simulink model "GradualClampTestslx"  (R2021b)
settings: Solver=FixedStepAuto  StartTime=0.0  StopTime=inf  RelTol=1e-3  EnableMultiTasking=on
libraries: vexarmcortexlib x23, simulink x8, vexcommonlib x2
settings Model: SimulationMode=external  NumberOfSteps=6  Creator=arago  LastModifiedBy=arago
settings DataIOCC: LimitDataPoints=on  SignalLoggingSaveFormat=ModelDataLogs  ReturnWorkspaceOutputs=off
settings OptimizationCC: ExpressionDepthLimit=2147483647  LifeSpan=Inf  MaxStackSize=64  EfficientTunableParamExpr=on
settings DebuggingCC: UnderspecifiedInitializationDetection=Classic  MergeDetectMultiDrivingBlocksExec=none  InheritedTsInSrcMsg=none  FcnCallInpInsideContextMsg=warning  UnconnectedInputMsg=none  UnconnectedOutputMsg=none  StateNameClashWarn=warning  SFUnexpectedBacktrackingDiag=warning  SFNoUnconditionalDefaultTransitionDiag=warning  SFExecutionAtInitializationDiag=none  SFMachineParentedDataDiag=warning  ArithmeticOperatorsInVariantConditions=warning
settings HardwareCC: ProdBitPerPointer=32  ProdBitPerSizeT=32  ProdBitPerPtrDiffT=32  ProdLargestAtomicInteger=Long  ProdLargestAtomicFloat=Double  ProdIntDivRoundTo=Undefined  ProdWordSize=32  ProdHWDeviceType=ARM Compatible->ARM Cortex
settings ModelReferenceCC: PropagateSignalLabelsOutOfModel=off
settings SFSimCC: MATLABDynamicMemAlloc=off  CustomCodeUndefinedFunction=UseInterfaceOnly
settings RTWCC: Description=Embedded Coder  SystemTargetFile=ert.tlc  HardwareBoard=ARM Cortex-based VEX Microcontroller  TemplateMakefile=ert_default_tmf  Toolchain=GNU Tools for VEX ARM Cortex
settings CodeAppCC: IgnoreCustomStorageClasses=off  CustomSymbolStrType=$N$R$M  StateflowObjectComments=on  InternalIdentifier=Classic
settings ERTTargetCC: CodeReplacementLibrary=GCC ARM Cortex-M3  MultiwordLength=2048  ConvertIfToSwitch=off  SuppressUnreachableDefaultCases=off

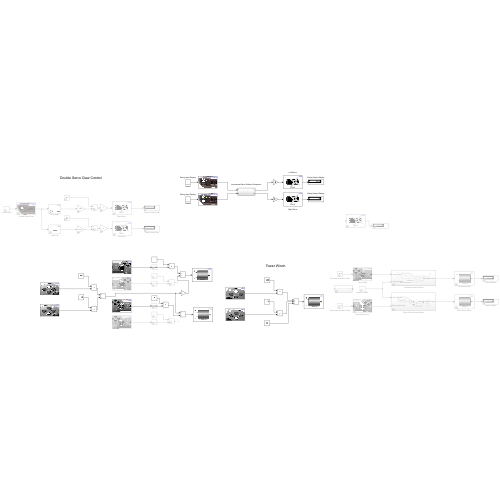
[thumbnail: Simulink's stored preview of the top-level diagram]
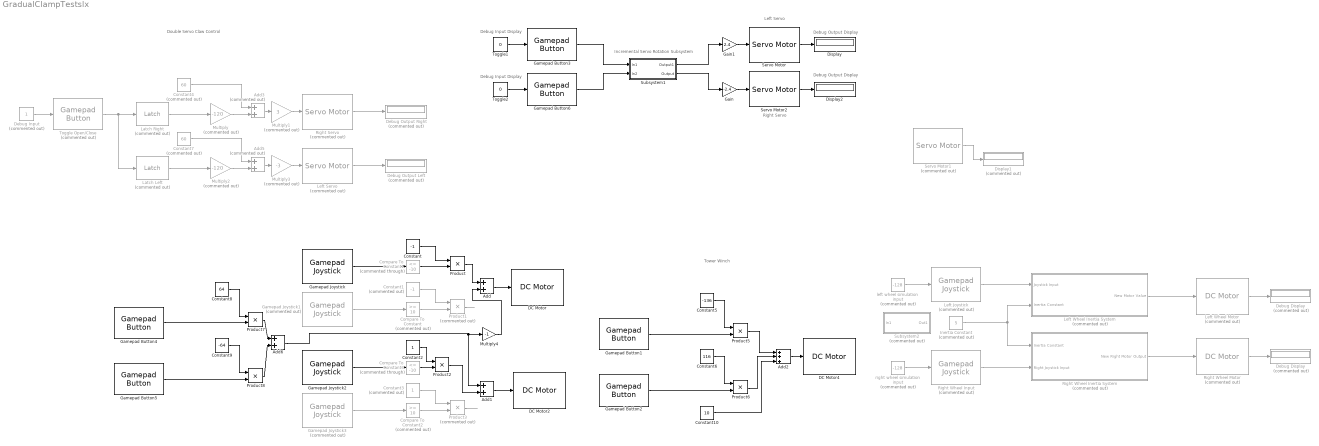
== system GradualClampTestslx ==
  note: Incremental Servo Rotation Subsystem
  note: Left Servo
  note: Double Servo Claw Control
  note: Tower Winch
  note: Right Servo
  note: Debug Output Display
  note: Debug Output Display
  note: Debug Input Display
  note: Debug Input Display
  " Debug Display" : Display  Commented=on
  Add : Sum
  Add1 : Sum
  Add2 : Sum  Inputs=+++
  Add3 : Sum  Commented=on
  Add5 : Sum  Commented=on
  Add6 : Sum
  Compare To Constant : simulink/Logic and Bit Operations/Compare To Constant  Commented=on  relop=>=  const=10  OutDataTypeStr=uint8
  Compare To Constant1 : simulink/Logic and Bit Operations/Compare To Constant  Commented=through  relop=<=  const=-10  OutDataTypeStr=uint8
  Compare To Constant2 : simulink/Logic and Bit Operations/Compare To Constant  Commented=on  relop=>=  const=10  OutDataTypeStr=uint8
  Compare To Constant3 : simulink/Logic and Bit Operations/Compare To Constant  Commented=through  relop=<=  const=-10  OutDataTypeStr=uint8
  Constant : Constant  Value=-1
  Constant1 : Constant  Commented=on  Value=-1
  Constant10 : Constant  Value=10
  Constant2 : Constant
  Constant3 : Constant  Commented=on
  Constant4 : Constant  Commented=on  Value=60
  Constant5 : Constant  Value=-136
  Constant6 : Constant  Value=116
  Constant7 : Constant  Commented=on  Value=60
  Constant8 : Constant  Value=64
  Constant9 : Constant  Value=-64
  DC Motor : vexarmcortexlib/Actuators/DC Motor  motor=2  scaleFactor=1/13.5  SimulationOut=off
      settings: SourceProductBaseCode=EC_VEX_MICRO
  DC Motor2 : vexarmcortexlib/Actuators/DC Motor  motor=3  scaleFactor=1/13.5  SimulationOut=off
      settings: SourceProductBaseCode=EC_VEX_MICRO
  DC Motor4 : vexarmcortexlib/Actuators/DC Motor  motor=6  scaleFactor=1/13.5  SimulationOut=off
      settings: SourceProductBaseCode=EC_VEX_MICRO
  Debug Display : Display  Commented=on
  Debug Input : Constant  Commented=on
      settings: OpenFcn=|
      | if strcmp('0',get_param(gcb, 'Value'))                        set_param(gcb, 'Value', '1');
      | else
      |             set_param(gcb, 'Value', '0');
      | end
  Debug Output Left : Display  Commented=on
  Debug Output Right : Display  Commented=on
  Display : Display
  Display1 : Display  Commented=on
  Display2 : Display
  Gain : Gain  Gain=-2.4
  Gain1 : Gain  Gain=2.4
  Gamepad Button1 : vexarmcortexlib/Gamepad/Gamepad Button  joystick=1  chan=8  button56=Up  button78=Up  SimulationIn=off  SampleTime=0.02
      settings: SourceProductBaseCode=EC_VEX_MICRO
  Gamepad Button2 : vexarmcortexlib/Gamepad/Gamepad Button  joystick=1  chan=8  button56=Up  button78=Down  SimulationIn=off  SampleTime=0.02
      settings: SourceProductBaseCode=EC_VEX_MICRO
  Gamepad Button3 : vexarmcortexlib/Gamepad/Gamepad Button  joystick=1  chan=6  button56=Up  button78=Down  SimulationIn=on  SampleTime=0.02
      settings: SourceProductBaseCode=EC_VEX_MICRO
  Gamepad Button4 : vexarmcortexlib/Gamepad/Gamepad Button  joystick=1  chan=7  button56=Up  button78=Up  SimulationIn=off  SampleTime=0.02
      settings: SourceProductBaseCode=EC_VEX_MICRO
  Gamepad Button5 : vexarmcortexlib/Gamepad/Gamepad Button  joystick=1  chan=7  button56=Up  button78=Down  SimulationIn=off  SampleTime=0.02
      settings: SourceProductBaseCode=EC_VEX_MICRO
  Gamepad Button6 : vexarmcortexlib/Gamepad/Gamepad Button  joystick=1  chan=6  button56=Down  button78=Down  SimulationIn=on  SampleTime=0.02
      settings: SourceProductBaseCode=EC_VEX_MICRO
  Gamepad Joystick : vexarmcortexlib/Gamepad/Gamepad Joystick  joystick=1  chan=2  SimulationIn=off  SampleTime=0.02
      settings: SourceProductBaseCode=EC_VEX_MICRO
  Gamepad Joystick1 : vexarmcortexlib/Gamepad/Gamepad Joystick  Commented=on  joystick=1  chan=2  SimulationIn=off  SampleTime=0.02
      settings: SourceProductBaseCode=EC_VEX_MICRO
  Gamepad Joystick2 : vexarmcortexlib/Gamepad/Gamepad Joystick  joystick=1  chan=3  SimulationIn=off  SampleTime=0.02
      settings: SourceProductBaseCode=EC_VEX_MICRO
  Gamepad Joystick3 : vexarmcortexlib/Gamepad/Gamepad Joystick  Commented=on  joystick=1  chan=3  SimulationIn=off  SampleTime=0.02
      settings: SourceProductBaseCode=EC_VEX_MICRO
  Inertia Constant : Constant  Commented=on  Value=5
  Latch Left : vexcommonlib/Latch  Commented=on  output0=off  BlockPlatform=vexarmcortex
      settings: SourceProductBaseCode=EC_VEX_MICRO,VEXV5
  Latch Right : vexcommonlib/Latch  Commented=on  output0=off  BlockPlatform=vexarmcortex
      settings: SourceProductBaseCode=EC_VEX_MICRO,VEXV5
  Left Joystick : vexarmcortexlib/Gamepad/Gamepad Joystick  Commented=on  joystick=1  chan=3  SimulationIn=on  SampleTime=0.02
      settings: SourceProductBaseCode=EC_VEX_MICRO
  Left Servo : vexarmcortexlib/Actuators/Servo Motor  Commented=on  motor=4  scaleFactor=60/127  SimulationOut=on
      settings: SourceProductBaseCode=EC_VEX_MICRO
  Left Wheel Inertia System : Subsystem  Commented=on
  Left Wheel Motor : vexarmcortexlib/Actuators/DC Motor  Commented=on  motor=2  scaleFactor=1/13.5  SimulationOut=on
      settings: SourceProductBaseCode=EC_VEX_MICRO
  Multiply : Gain  Commented=on  Gain=-120
  Multiply1 : Gain  Commented=on  Gain=3
  Multiply2 : Gain  Commented=on  Gain=-120
  Multiply3 : Gain  Commented=on  Gain=-3
  Multiply4 : Gain  Gain=-1
  Product{,2,5..8} (6 alike) : Product
  Product1 : Product  Commented=on
  Product3 : Product  Commented=on
  Right Servo : vexarmcortexlib/Actuators/Servo Motor  Commented=on  motor=5  scaleFactor=60/127  SimulationOut=on
      settings: SourceProductBaseCode=EC_VEX_MICRO
  Right Wheel Inertia System : Subsystem  Commented=on
  Right Wheel Input : vexarmcortexlib/Gamepad/Gamepad Joystick  Commented=on  joystick=1  chan=2  SimulationIn=on  SampleTime=0.02
      settings: SourceProductBaseCode=EC_VEX_MICRO
  Right Wheel Motor : vexarmcortexlib/Actuators/DC Motor  Commented=on  motor=3  scaleFactor=1/13.5  SimulationOut=on
      settings: SourceProductBaseCode=EC_VEX_MICRO
  Servo Motor : vexarmcortexlib/Actuators/Servo Motor  motor=5  scaleFactor=60/127  SimulationOut=on
      settings: SourceProductBaseCode=EC_VEX_MICRO
  Servo Motor1 : vexarmcortexlib/Actuators/Servo Motor  Commented=on  motor=5  scaleFactor=60/127  SimulationOut=on
      settings: SourceProductBaseCode=EC_VEX_MICRO
  Servo Motor2 : vexarmcortexlib/Actuators/Servo Motor  motor=4  scaleFactor=60/127  SimulationOut=on
      settings: SourceProductBaseCode=EC_VEX_MICRO
  Subsystem1 : Subsystem
  Subsystem2 : Subsystem  Commented=on
  Toggle Open/Close : vexarmcortexlib/Gamepad/Gamepad Button  Commented=on  joystick=1  chan=6  button56=Up  button78=Down  SimulationIn=on  SampleTime=0.02
      settings: SourceProductBaseCode=EC_VEX_MICRO
  Toggle1 : Constant  Value=0
      settings: OpenFcn=|
      | if strcmp('0',get_param(gcb, 'Value'))                        set_param(gcb, 'Value', '1');
      | else
      |             set_param(gcb, 'Value', '0');
      | end
  Toggle2 : Constant  Value=0
      settings: OpenFcn=|
      | if strcmp('0',get_param(gcb, 'Value'))                        set_param(gcb, 'Value', '1');
      | else
      |             set_param(gcb, 'Value', '0');
      | end
  left wheel simulation input : Constant  Commented=on  Value=-128  SampleTime=0.02
  right wheel simulation input : Constant  Commented=on  Value=-128  SampleTime=0.02
  wires:
  Gamepad Joystick1/1 -> Compare To Constant/1
  Gamepad Joystick/1 -> Compare To Constant1/1
  Compare To Constant/1 -> Product1/2
  Compare To Constant1/1 -> Product/2
  Constant/1 -> Product/1
  Constant1/1 -> Product1/1
  Constant2/1 -> Product2/1
  Constant3/1 -> Product3/1
  Gamepad Joystick2/1 -> Compare To Constant3/1
  Compare To Constant3/1 -> Product2/2
  Product3/1 -> ?
  Product2/1 -> Add1/2
  Compare To Constant2/1 -> Product3/2
  Gamepad Joystick3/1 -> Compare To Constant2/1
  Toggle Open/Close/1 -> Latch Left/1, Latch Right/1
  Latch Right/1 -> Multiply/1
  Constant4/1 -> Add3/1
  Gamepad Button1/1 -> Product5/2
  Constant5/1 -> Product5/1
  Product5/1 -> Add2/1
  Product6/1 -> Add2/2
  Constant6/1 -> Product6/1
  Gamepad Button2/1 -> Product6/2
  Add/1 -> DC Motor/1
  Product/1 -> Add/1
  Product1/1 -> ?
  Add1/1 -> DC Motor2/1
  Add2/1 -> DC Motor4/1
  Debug Input/1 -> Toggle Open/Close/1
  Servo Motor/1 -> Display/1
  Multiply/1 -> Add3/2
  Add3/1 -> Multiply1/1
  Toggle1/1 -> Gamepad Button3/1
  Gamepad Button3/1 -> Subsystem1/1(In1)
  Servo Motor1/1 -> Display1/1
  Constant7/1 -> Add5/1
  Multiply2/1 -> Add5/2
  Latch Left/1 -> Multiply2/1
  Servo Motor2/1 -> Display2/1
  Add5/1 -> Multiply3/1
  Add6/1 -> Multiply4/1, Add1/1
  Gamepad Button5/1 -> Product8/2
  Product7/1 -> Add6/1
  Product8/1 -> Add6/2
  Gamepad Button4/1 -> Product7/2
  Constant9/1 -> Product8/1
  Constant8/1 -> Product7/1
  Multiply4/1 -> Add/2
  Subsystem1/1(Output1) -> Gain1/1
  Subsystem1/2(Output) -> Gain/1
  Toggle2/1 -> Gamepad Button6/1
  Gamepad Button6/1 -> Subsystem1/2(In2)
  Left Wheel Motor/1 -> " Debug Display"/1
  right wheel simulation input/1 -> Right Wheel Input/1
  Right Wheel Inertia System/1(New Right Motor Output) -> Right Wheel Motor/1
  left wheel simulation input/1 -> Left Joystick/1
  Right Wheel Motor/1 -> Debug Display/1
  Left Wheel Inertia System/1(New Motor Value) -> Left Wheel Motor/1
  Right Wheel Input/1 -> Right Wheel Inertia System/2(Right Joystick Input)
  Inertia Constant/1 -> Right Wheel Inertia System/1(Inertia Constant), Left Wheel Inertia System/2(Inertia Constant)
  Left Joystick/1 -> Left Wheel Inertia System/1(Joystick Input)
  Gain/1 -> Servo Motor2/1
  Gain1/1 -> Servo Motor/1
  Right Servo/1 -> Debug Output Right/1
  Left Servo/1 -> Debug Output Left/1
  Multiply1/1 -> Right Servo/1
  Multiply3/1 -> Left Servo/1
  Constant10/1 -> Add2/3

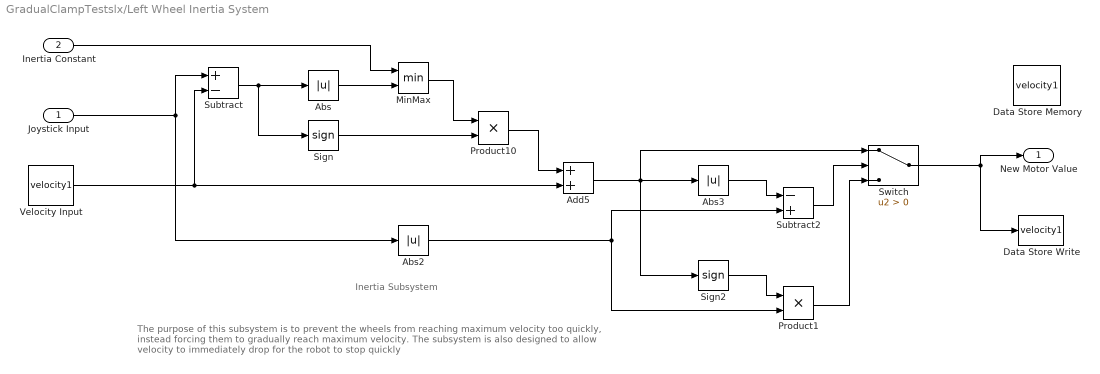
== system GradualClampTestslx/Left Wheel Inertia System ==
  note: The purpose of this subsystem is to prevent the wheels from reaching maximum velocity too quickly, instead forcing them to gradually reach maximum velocity. The subsystem is also designed to allow velocity to immediately drop for the robot to stop quickly
  note: Inertia Subsystem
  Joystick Input : Inport
  Inertia Constant : Inport  Port=2
  Abs : Abs
  Abs2 : Abs
  Abs3 : Abs
  Add5 : Sum
  Data Store Memory : DataStoreMemory  DataStoreName=velocity1  ReadBeforeWriteMsg=warning  WriteAfterWriteMsg=warning  WriteAfterReadMsg=warning  ShowAdditionalParam=off
  Data Store Write : DataStoreWrite  DataStoreName=velocity1  SampleTime=0.02  IndexOptions=Index vector (dialog)  Indices=1  OutputSizes=1
  MinMax : MinMax  Inputs=2
  Product1 : Product  RndMeth=Zero
  Product10 : Product  RndMeth=Zero
  Sign : Signum
  Sign2 : Signum
  Subtract : Sum  Inputs=+-
  Subtract2 : Sum  Inputs=-+
  Switch : Switch  Criteria=u2 > Threshold
  Velocity Input : DataStoreRead  DataStoreName=velocity1  SampleTime=0.02  IndexOptions=Index vector (dialog)  Indices=1  OutputSizes=1
  New Motor Value : Outport
  wires:
  Joystick Input/1 -> Subtract/1, Abs2/1
  Subtract/1 -> Sign/1, Abs/1
  Add5/1 -> Sign2/1, Switch/1, Abs3/1
  Abs/1 -> MinMax/2
  Sign/1 -> Product10/2
  Velocity Input/1 -> Subtract/2, Add5/2
  Abs2/1 -> Subtract2/2, Product1/2
  Product10/1 -> Add5/1
  Sign2/1 -> Product1/1
  MinMax/1 -> Product10/1
  Inertia Constant/1 -> MinMax/1
  Switch/1 -> New Motor Value/1, Data Store Write/1
  Subtract2/1 -> Switch/2
  Abs3/1 -> Subtract2/1
  Product1/1 -> Switch/3

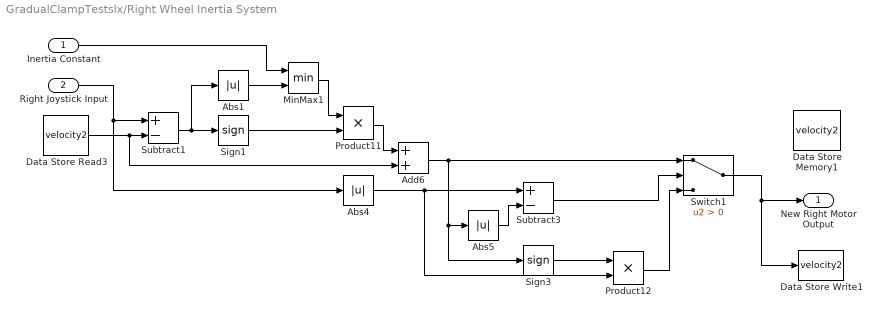
== system GradualClampTestslx/Right Wheel Inertia System ==
  Inertia Constant : Inport
  Right Joystick Input : Inport  Port=2
  Abs1 : Abs
  Abs4 : Abs
  Abs5 : Abs
  Add6 : Sum
  Data Store Memory1 : DataStoreMemory  DataStoreName=velocity2  ReadBeforeWriteMsg=warning  WriteAfterWriteMsg=warning  WriteAfterReadMsg=warning  ShowAdditionalParam=off
  Data Store Read3 : DataStoreRead  DataStoreName=velocity2  SampleTime=0.02  IndexOptions=Index vector (dialog)  Indices=1  OutputSizes=1
  Data Store Write1 : DataStoreWrite  DataStoreName=velocity2  SampleTime=0.02  IndexOptions=Index vector (dialog)  Indices=1  OutputSizes=1
  MinMax1 : MinMax  Inputs=2
  Product11 : Product  RndMeth=Zero
  Product12 : Product  RndMeth=Zero
  Sign1 : Signum
  Sign3 : Signum
  Subtract1 : Sum  Inputs=+-
  Subtract3 : Sum  Inputs=+-
  Switch1 : Switch  Criteria=u2 > Threshold
  New Right Motor Output : Outport
  wires:
  MinMax1/1 -> Product11/1
  Abs5/1 -> Subtract3/2
  Product11/1 -> Add6/1
  Abs4/1 -> Product12/2, Subtract3/1
  Abs1/1 -> MinMax1/2
  Subtract3/1 -> Switch1/2
  Subtract1/1 -> Abs1/1, Sign1/1
  Sign1/1 -> Product11/2
  Sign3/1 -> Product12/1
  Data Store Read3/1 -> Subtract1/2, Add6/2
  Add6/1 -> Abs5/1, Sign3/1, Switch1/1
  Right Joystick Input/1 -> Abs4/1, Subtract1/1
  Inertia Constant/1 -> MinMax1/1
  Product12/1 -> Switch1/3
  Switch1/1 -> Data Store Write1/1, New Right Motor Output/1

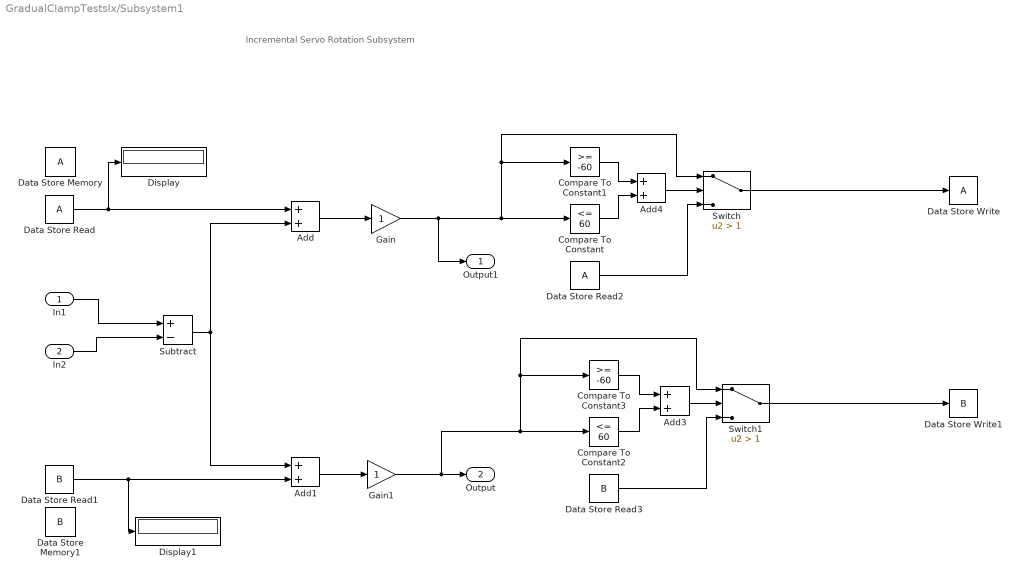
== system GradualClampTestslx/Subsystem1 ==
  note: Incremental Servo Rotation Subsystem
  In1 : Inport
  In2 : Inport  Port=2
  Add{,1,3..4} (4 alike) : Sum
  Compare To Constant : simulink/Logic and Bit Operations/Compare To Constant  relop=<=  const=60  OutDataTypeStr=boolean
  Compare To Constant1 : simulink/Logic and Bit Operations/Compare To Constant  relop=>=  const=-60  OutDataTypeStr=boolean
  Compare To Constant2 : simulink/Logic and Bit Operations/Compare To Constant  relop=<=  const=60  OutDataTypeStr=boolean
  Compare To Constant3 : simulink/Logic and Bit Operations/Compare To Constant  relop=>=  const=-60  OutDataTypeStr=boolean
  Data Store Memory : DataStoreMemory  ReadBeforeWriteMsg=warning  WriteAfterWriteMsg=warning  WriteAfterReadMsg=warning  ShowAdditionalParam=off
  Data Store Memory1 : DataStoreMemory  DataStoreName=B  ReadBeforeWriteMsg=warning  WriteAfterWriteMsg=warning  WriteAfterReadMsg=warning  ShowAdditionalParam=off
  Data Store Read : DataStoreRead  IndexOptions=Index vector (dialog)  Indices=1  OutputSizes=1
  Data Store Read1 : DataStoreRead  DataStoreName=B  IndexOptions=Index vector (dialog)  Indices=1  OutputSizes=1
  Data Store Read2 : DataStoreRead  IndexOptions=Index vector (dialog)  Indices=1  OutputSizes=1
  Data Store Read3 : DataStoreRead  DataStoreName=B  IndexOptions=Index vector (dialog)  Indices=1  OutputSizes=1
  Data Store Write : DataStoreWrite  IndexOptions=Index vector (dialog)  Indices=1  OutputSizes=1
  Data Store Write1 : DataStoreWrite  DataStoreName=B  IndexOptions=Index vector (dialog)  Indices=1  OutputSizes=1
  Display : Display
  Display1 : Display
  Gain : Gain
  Gain1 : Gain
  Subtract : Sum  Inputs=+-
  Switch : Switch  Criteria=u2 > Threshold  Threshold=1
  Switch1 : Switch  Criteria=u2 > Threshold  Threshold=1
  Output1 : Outport
  Output : Outport  Port=2
  wires:
  In1/1 -> Subtract/1
  Add/1 -> Gain/1
  Add1/1 -> Gain1/1
  In2/1 -> Subtract/2
  Subtract/1 -> Add1/1, Add/2
  Gain/1 -> Compare To Constant1/1, Switch/1, Compare To Constant/1, Output1/1
  Switch/1 -> Data Store Write/1
  Switch1/1 -> Data Store Write1/1
  Data Store Read/1 -> Display/1, Add/1
  Data Store Read1/1 -> Display1/1, Add1/2
  Compare To Constant1/1 -> Add4/1
  Compare To Constant/1 -> Add4/2
  Add4/1 -> Switch/2
  Data Store Read2/1 -> Switch/3
  Compare To Constant2/1 -> Add3/2
  Data Store Read3/1 -> Switch1/3
  Add3/1 -> Switch1/2
  Compare To Constant3/1 -> Add3/1
  Gain1/1 -> Compare To Constant3/1, Switch1/1, Compare To Constant2/1, Output/1

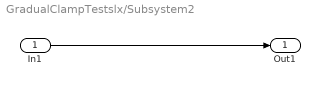
== system GradualClampTestslx/Subsystem2 ==
  In1 : Inport
  Out1 : Outport
  wires:
  In1/1 -> Out1/1
